simulink model "rcams"  (R2024b)
settings: Solver=VariableStepAuto  StartTime=0.0  StopTime=TF  RelTol=1e-3
values from neighbouring files (symbols this model uses):
  x0 = [0 ... (first row only)    [initialiseGEODETIC.m]
undefined symbols (not defined in the file or in its folder): RCAM_model
settings Model: Creator=varsh  LastModifiedBy=varsh
settings DataIOCC: SaveFormat=StructureWithTime  SaveState=on

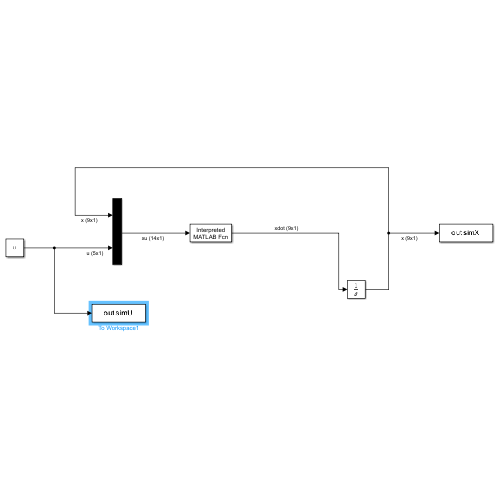
[thumbnail: Simulink's stored preview of the top-level diagram]
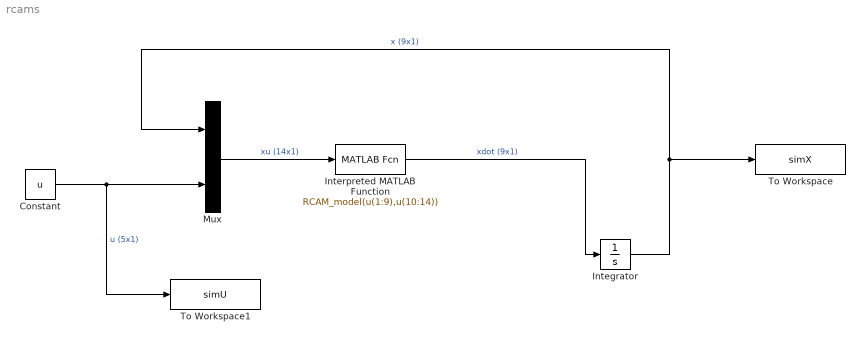
== system rcams ==
  Constant : Constant  Value=u
  Integrator : Integrator  InitialCondition=x0
  Interpreted MATLAB Function : MATLABFcn  MATLABFcn=RCAM_model(u(1:9),u(10:14))
  Mux : Mux  Inputs=2
  To Workspace : ToWorkspace  VariableName=simX  SaveFormat=Timeseries  SampleTime=-1
  To Workspace1 : ToWorkspace  VariableName=simU  SaveFormat=Timeseries  SampleTime=-1
  wires:
  Interpreted MATLAB Function/1 -> Integrator/1  "xdot (9x1)"
  Integrator/1 -> To Workspace/1, Mux/1  "x (9x1)"
  Constant/1 -> To Workspace1/1, Mux/2  "u (5x1)"
  Mux/1 -> Interpreted MATLAB Function/1  "xu (14x1)"
